simulink model "FFT4dSpace_rtKolloq"  (R2021a)
settings: Solver=FixedStepDiscrete  StartTime=0.0  StopTime=0.01  FixedStep=1e-5 % Ts  RelTol=1e-3
values from neighbouring files (symbols this model uses):
  NFFT2 = 2^10    (= 1024)    [FFT4dSpace_rtKolloq_1_i.m]    (also in FFT4dSpace_rtKolloq_i.m)
  Ts = 1e-3    (= 0.001)    [FFT4dSpace_rtKolloq_1_i.m]    (also in FFT4dSpace_rtKolloq_i.m)
undefined symbols (not defined in the file or in its folder): mdlPara
libraries: dspxfrm3 x1, dspsigops x1
settings Model: Creator=nitr  LastModifiedBy=nitr

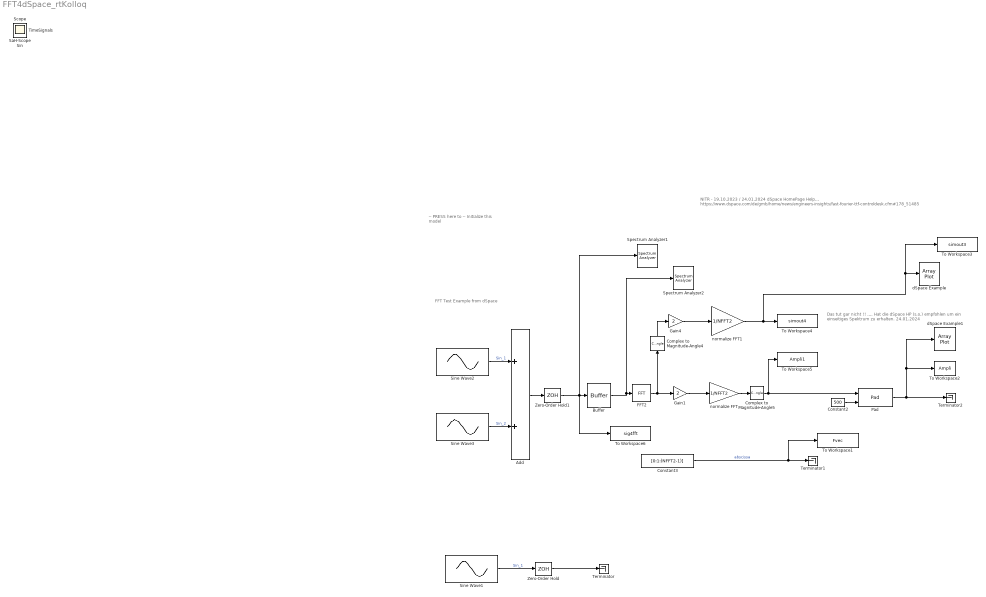
== system FFT4dSpace_rtKolloq ==
  note: Das tut gar nicht !! ....
      | Hat die dSpace HP (s.o.) empfohlen um
      | ein einseitiges Spektrum zu erhalten.
      |
      | 24.01.2024
  note: NITR - 19.10.2023 / 24.01.2024
      |
      | dSpace HomePage Help...
      | https://www.dspace.com/de/gmb/home/news/engineers-insights/fast-fourier-ttf-controldesk.cfm#178_51485
  note: -- PRESS here to --
      | Initialize this model
  note: FFT Test Example from dSpace
  Add : Sum
  Buffer : Buffer  N=NFFT2  OutputFrames=off
  Complex to Magnitude-Angle4 : ComplexToMagnitudeAngle  Output=Magnitude
  Complex to Magnitude-Angle5 : ComplexToMagnitudeAngle  Output=Magnitude
  Constant2 : Constant  Value=500
  Constant3 : Constant  Value=[0:1:(NFFT2-1)]
  FFT2 : dspxfrm3/FFT  FFTImplementation=Auto  CompMethod=Table lookup  TableOpt=NEW  TableOptActive=Speed  BitRevOrder=off  Normalize=off  InheritFFTLength=off  FFTLength=NFFT2  WrapInput=on  roundingMode=Floor  overflowMode=off  firstCoeffDataTypeStr=Inherit: Same word length as input  firstCoeffLastDataTypeStr=Inherit: Same word length as input  outputMin=[]  outputMax=[]
  Gain1 : Gain  Gain=2
  Gain4 : Gain  Gain=2
  Pad : dspsigops/Pad  padAlong=Columns  dimsToPad=1  valSrc=Input port  padVal=0  spec=Output size  padNumOutRowsSpecMethod=User-specified  numOutRows=NFFT2  padNumOutColsSpecMethod=User-specified  numOutCols=1  isVarDimsMode=off  padBeginning=0  padEnd=0  outSizeMode=User-specified  outSize=1  padSigAt=End  trunc_flag=None  roundingMode=Floor  overflowMode=off  truncOrWrapMode=Truncate  wrap_flag=None
      settings: SourceProductBaseCode=DS
  Sine Wave1 : Sin  Amplitude=mdlPara.a1  Bias=mdlPara.Bias1  Frequency=mdlPara.om1  SampleTime=0
  Sine Wave2 : Sin  Amplitude=mdlPara.a1  Bias=mdlPara.Bias1  Frequency=mdlPara.om1  SampleTime=0
  Sine Wave3 : Sin  Amplitude=mdlPara.a2  Bias=mdlPara.Bias2  Frequency=mdlPara.om2  SampleTime=0
  Spectrum Analyzer1 : SpectrumAnalyzer
  Spectrum Analyzer2 : SpectrumAnalyzer
  Terminator : Terminator
  Terminator1 : Terminator
  Terminator2 : Terminator
  To Workspace1 : ToWorkspace  VariableName=Fvec  SampleTime=-1
  To Workspace2 : ToWorkspace  VariableName=Ampli  SampleTime=-1
  To Workspace3 : ToWorkspace  VariableName=simout3  SampleTime=-1
  To Workspace4 : ToWorkspace  VariableName=simout4  SampleTime=-1
  To Workspace5 : ToWorkspace  VariableName=Ampli1  SampleTime=-1
  To Workspace6 : ToWorkspace  VariableName=sig4fft  SaveFormat=Structure With Time  SampleTime=Ts
  Zero-Order Hold : ZeroOrderHold  SampleTime=Ts
  Zero-Order Hold1 : ZeroOrderHold  SampleTime=Ts
  dSpace Example : ArrayPlot  WindowPosition=[854 513 800 435]  SampleIncrement=1000/128  XOffset=-500  CustomXData=[-500+500/128:1000/128:500]  PlotType=Line  AxesScaling=Manual  YLimits=[-7.69577,71.9475]  DefaultConfigurationName=dsp.scopes.ArrayPlotBlockSpecification
  dSpace Example1 : ArrayPlot  WindowPosition=[64.000000,264.000000,702.000000,531.000000,]  Visible=on  XDataMode=Custom  SampleIncrement=1000/128  XOffset=-500  CustomXData=[-500+500/128:1000/128:500]  PlotType=Line  AxesScaling=Manual  YLimits=[-7.69577,71.9475]  DefaultConfigurationName=dsp.scopes.ArrayPlotBlockSpecification
  normalize FFT : Gain  Gain=1/NFFT2
  normalize FFT1 : Gain  Gain=1/NFFT2
  SaH-Scope : Scope
  Scope : Scope
  Sin : Scope
  TimeSignals : Scope
  wires:
  Constant3/1 -> To Workspace1/1, Terminator1/1  "abscissa"
  Pad/1 -> dSpace Example1/1, To Workspace2/1, Terminator2/1
  Constant2/1 -> Pad/2
  Buffer/1 -> Spectrum Analyzer2/1, FFT2/1
  Gain1/1 -> normalize FFT/1
  Sine Wave3/1 -> Add/2  "Sin_2"
  Sine Wave2/1 -> Add/1  "Sin_1"
  Add/1 -> Zero-Order Hold1/1
  normalize FFT1/1 -> To Workspace3/1, dSpace Example/1, To Workspace4/1
  Complex to Magnitude-Angle4/1 -> Gain4/1
  Gain4/1 -> normalize FFT1/1
  normalize FFT/1 -> Complex to Magnitude-Angle5/1
  FFT2/1 -> Complex to Magnitude-Angle4/1, Gain1/1
  Complex to Magnitude-Angle5/1 -> To Workspace5/1, Pad/1
  Sine Wave1/1 -> Zero-Order Hold/1  "Sin_1"
  Zero-Order Hold/1 -> Terminator/1
  Zero-Order Hold1/1 -> Buffer/1, Spectrum Analyzer1/1, To Workspace6/1
